simulink model "V2X_Core_SRI_coding_rate_symbol"  (R2023b)
settings: Solver=ode23tb  StartTime=0.0  StopTime=50  MaxStep=1e-2  RelTol=1e-3  AbsTol=1e-3
StopFcn:
  | run('saving.m')
values from neighbouring files (symbols this model uses):
  b = 1.6    [a2024_v2x_matlab_6veh.m]
  m = 2000    [a2024_v2x_matlab_6veh.m]
  mEgo = 1500    [a2024_v2x_matlab_6veh.m]
  Mode = 1    [a2024_v2x_matlab_6veh.m]    (also in v2x_matlab.m; v2x_matlabV2.m; v2x_matlab_6veh.m; v2x_matlab_R.m)
  RefSpeed = 90/3.6    (= 25)    [v2x_matlabV2.m]    (also in v2x_matlab_R.m)
  RelDistThreshold = 300    [v2x_matlabV2.m]    (also in v2x_matlab_R.m)
  s = RandStream("dsfmt19937","Seed",15)    [v2x_matlab.m]
  sampleTime = 0.1    [a2024_v2x_matlab_6veh.m]    (also in v2x_matlab.m; v2x_matlabV2.m; v2x_matlab_6veh.m; v2x_matlab_R.m)
  waypoints = [egoWP(:,2) egoWP(:,1), zeroforwp]    [a2024_v2x_matlab_6veh.m]    (also in misc.m = data.data.ActorSpecifications(1,1).Waypoints(:,[1,2]); v2x_matlab.m = data.data.ActorSpecifications(1,1).Waypoints(:,[1,2]); v2x_matlabV2.m = [5 -1.6 0; v2x_matlab_R.m = [5 -1.6 0)
  ZeroActors = struct(     'ActorID',0,     'Position', [1000 1000 1000],      'Velocity', [0 0 0],      'Roll', 0,      'Pitch', 0,      'Yaw', 0,      'AngularVelocity', [0 0 0])    [v2x_matlabV2.m]    (also in v2x_matlab_R.m)
undefined symbols (not defined in the file or in its folder): Battery, Brakes, Control, DiscIntNeverNeededParam, doppler, Drivetrain, ElectricMotor, Env, FB_flag, Init, SNR_value_list, Vehicle, Wheels
libraries: simulink x45, commofdm x29, commdigbbndam3 x15, commchan3 x14, simulink_extras x13, commcnvcod2 x12, commdigbbndpm3 x11, commblkintrlv2 x10, dspmathops x6, sharedtransform x6, autolibutils x6, autolibsharedcoupling x4
(part 2 of 8)

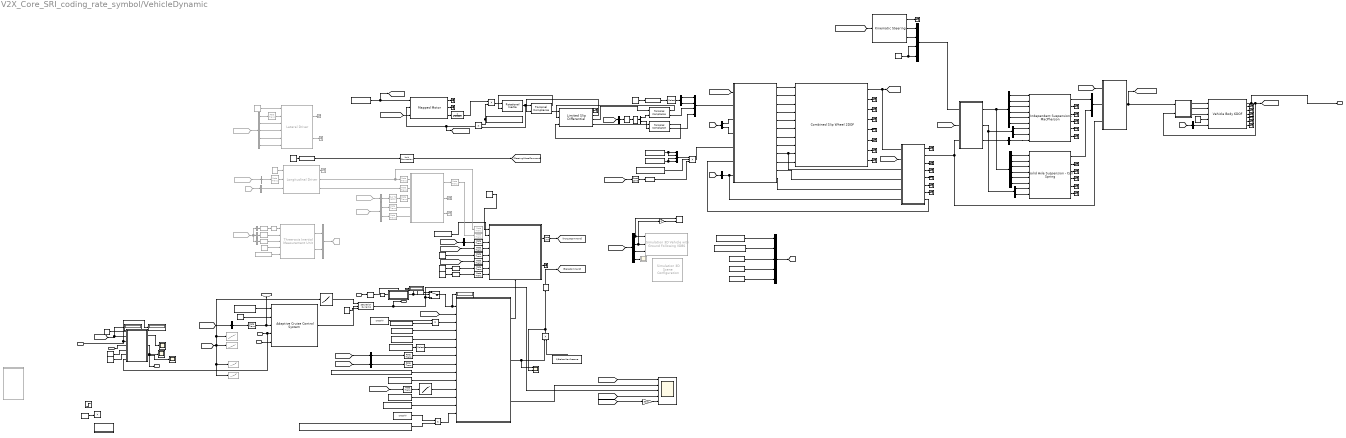
== system V2X_Core_SRI_coding_rate_symbol/VehicleDynamic ==
  note: ACC
  note: ENVIRONMENT
  note: CHASSIS
  note: VISAULS
  note: DRIVER INPUT
  note: WHEELS
  note: SUSPENSION
  note: STEERING
  note: ELECTRIC
  note: SENSOR
  note: BRAKE HYDRAULICS
  note: CONTROL
  note: DRIVETRAIN
  note: SRI
  u : Inport
  PDR : Inport  Port=2
  RelDist : Inport  Port=3
  RelativeVelocity : Inport  Port=4
  TTC : Inport  Port=5
  1-D Lookup Table : Lookup_n-D  NumberOfTableDimensions=1  BreakpointsForDimension1=ElectricMotor.SpeedVector  Table=ElectricMotor.TorqueVector  InternalRulePriority=Speed  RndMeth=Simplest
  1-D Lookup Table1 : Lookup_n-D  NumberOfTableDimensions=1  BreakpointsForDimension1=[0;5;15]  Table=[1;1.2;4]  InternalRulePriority=Speed  RndMeth=Simplest
  AccelerationToTrq : Subsystem
  Adaptive Cruise Control System1 : mpcadaslib/Adaptive Cruise Control System  EgoModel=tf([0.335,0.5],[0.3,0.7,0])  InitialEgoVelocity=Init.VelocityVector(1)  DefaultSpacing=10  MaxVelocity=60  MinAcceleration=-2  amin_ext=off  MaxAcceleration=4  amax_ext=off  Ts=0.1  PredictionHorizon=50  ControllerBehavior=0.950  suboptimal=off  maxiter=10  datatypeopt=double  optmode=off  trackmode=off
      settings: LibrarySourceBlock=mpclib/Automated Driving/Adaptive Cruise Control System
  Bus Creator : BusCreator  Inputs=2
  Bus Creator1 : BusCreator  Commented=on  Inputs=2
  Bus Creator2 : BusCreator  Inputs=5
  Bus Selector : BusSelector  OutputSignals=Front.zFront,Front.ReFront,Front.zdotFront,Front.FxFront,Front.FyFront,Front.MFront
  Bus Selector1 : BusSelector  Commented=on  OutputSignals=Omega,BrkPrs
  Bus Selector10 : BusSelector  OutputSignals=Omega
  Bus Selector11 : BusSelector  OutputSignals=BdyFrm.Cg.Vel.xdot
  Bus Selector12 : BusSelector  OutputSignals=Ground,Friction
  Bus Selector13 : BusSelector  OutputSignals=DCM
  Bus Selector14 : BusSelector  OutputSignals=WindXYZ
  Bus Selector15 : BusSelector  OutputSignals=InertFrm.Cg.Disp.X,InertFrm.Cg.Disp.Y,InertFrm.Cg.Ang.psi,BdyFrm.Cg.Vel.xdot
  Bus Selector16 : BusSelector  Commented=on  OutputSignals=Grade
  Bus Selector17 : BusSelector  Commented=on  OutputSignals=BdyFrm.Cg.Vel.xdot
  Bus Selector18 : BusSelector  Commented=on  OutputSignals=BdyFrm.Cg.Vel.xdot,InertFrm.Cg.Disp.Y,BdyFrm.Cg.Vel.ydot,InertFrm.Cg.Ang.psi,BdyFrm.Cg.AngVel.r
  Bus Selector19 : BusSelector  OutputSignals=BdyFrm.Cg.Vel.xdot
  Bus Selector2 : BusSelector  Commented=on  OutputSignals=BdyFrm.Cg.Acc.ax,BdyFrm.Cg.Acc.ay,BdyFrm.Cg.Acc.az  OutputAsBus=on
  Bus Selector20 : BusSelector  OutputSignals=Mx  OutputAsBus=on
  Bus Selector21 : BusSelector  OutputSignals=BdyFrm.Forces.Drag.Fx
  Bus Selector3 : BusSelector  OutputSignals=Front.VehPFront,Front.VehVFront
  Bus Selector4 : BusSelector  OutputSignals=Rear.VehPRear,Rear.VehVRear
  Bus Selector5 : BusSelector  Commented=on  OutputSignals=BdyFrm.Cg.AngVel.p,BdyFrm.Cg.AngVel.q,BdyFrm.Cg.AngVel.r  OutputAsBus=on
  Bus Selector6 : BusSelector  Commented=on  OutputSignals=BdyFrm.Cg.AngAcc.pdot,BdyFrm.Cg.AngAcc.qdot,BdyFrm.Cg.AngAcc.rdot  OutputAsBus=on
  Bus Selector7 : BusSelector  OutputSignals=Rear.zRear,Rear.ReRear,Rear.zdotRear,Rear.FxRear,Rear.FyRear,Rear.MRear
  Bus Selector8 : BusSelector  Commented=on  OutputSignals=BdyFrm.Cg.Acc.xddot,BdyFrm.Cg.Acc.yddot,BdyFrm.Cg.Acc.zddot  OutputAsBus=on
  Bus Selector9 : BusSelector  OutputSignals=StrgAngFront
  Bus to Vector{,1..3} (4 alike) : BusToVector  Commented=on
  Clock : simulink_extras/Flip Flops/Clock  period=sampleTime
  Combined Slip Wheel 2DOF : vehdynlibtire/Combined Slip Wheel 2DOF  tireType=Light passenger car 205/60R15  BrakeType=Disc  vertType=Magic Formula  plySteer=off  turnslip=off  mu_static=ones(1,4) .* Brakes.StaticFrictionCoeff  mu_kinetic=ones(1,4) .* Brakes.KineticFrictionCoeff  disk_abore=ones(1,4) .* Brakes.DiskBore  Rm=ones(1,4) .* Brakes.BrakePadMeanRadius  num_pads=ones(1,4) .* Brakes.NumPads  drum_abore=0.0508  drum_a=0.123  drum_c=0.212  drum_r=0.15  drum_theta1=0  drum_theta2=126  brake_p_bpt=[1 11.4736842105263 21.9473684210526 32.4210526315789 42.8947368421053 53.3684210526316 63.8421052631579 74.3157894736842 84.7894736842105 95.2631578947368 105.736842105263 116.210526315789 126.684210526316 137.157894736842 147.631578947368 158.105263157895 168.578947368421 179.052631578947 189.526315789474 200]  brake_n_bpt=[0 52.6315789473684 105.263157894737 157.894736842105 210.526315789474 263.157894736842 315.789473684211 368.421052631579 421.052631578947 473.684210526316 526.315789473684 578.947368421053 631.578947368421 684.210526315789 736.842105263158 789.473684210526 842.105263157895 894.736842105263 947.368421052632 1000]  f_brake_t=[43.4900602404453 42.5056030554862 41.5350898940194 40.5780454442085 39.6340111501808 38.7025443887544 37.7832176914519 36.8756180088306 35.9793460143796 35.0940154454303 34.2192524787115 33.3546951383474 32.4999927342521 31.6548053290159 30.8188032315107 29.991666515561 29.1730845621415 28.362755623661 27.5603864089927 26.765691687993;498.991217495636 487.695866636631 476.560505099801 465.579679307235 454.748127933653 444.060772460445 433.51270824929 423.099196101319 412.81565427025 402.657650900201 392.620896861006 382.701238955775 372.894653477208 363.197240090814 353.605216024701 344.114910546964 334.722759712992 325.425301366216 316.219170376863 307.10109410434;954.492374750826 932.886130217776 911.585920305583 890.581313170261 869.862244717126 849.419000532136 829.242198807128 809.322774193808 789.651962526121 770.221286354971 751.0225412433 732.047782773203 713.289314220164 694.739674852612 676.391628817892 658.238154578366 640.272434863842 622.48784710877 604.877954344734 587.436496520688;1409.99353200602 1378.07639379892 1346.61133551136 1315.58294703329 1284.9763615006 1254.77722860383 1224.97168936497 1195.5463522863 1166.48827078199 1137.78492180974 1109.42418562559 1081.39432659063 1053.68397496312 1026.28210961441 999.178041611083 972.361398609768 945.822110014692 919.550392851325 893.536738312604 867.771898937035;1865.49468926121 1823.26665738007 1781.63675071715 1740.58458089631 1700.09047828407 1660.13545667552 1620.7011799228 1581.76993037878 1543.32457903786 1505.34855726451 1467.82583000789 1430.74087040806 1394.07863570608 1357.82454437621 1321.96445440427 1286.48464264117 1251.37178516554 1216.61293859388 1182.19552228048 1148.10730135338;2320.9958465164 2268.45692096121 2216.66216592293 2165.58621475934 2115.20459506754 2065.49368474721 2016.43067048064 1967.99350847127 1920.16088729373 1872.91219271928 1826.22747439018 1780.08741422549 1734.47329644903 1689.36697913801 1644.75086719747 1600.60788667257 1556.92146031639 1513.67548433643 1470.85430624835 1428.44270376973;2776.49700377159 2713.64718454235 2651.68758112871 2590.58784862237 2530.31871185102 2470.8519128189 2412.16016103848 2354.21708656376 2296.9971955496 2240.47582817405 2184.62911877248 2129.43395804292 2074.86795719199 2020.9094138998 1967.53727999066 1914.73113070398 1862.47113546724 1810.73803007899 1759.51309021622 1708.77810618608;3231.99816102678 3158.8374481235 3086.71299633449 3015.58948248539 2945.43282863449 2876.21014089059 2807.88965159632 2740.44066465625 2673.83350380547 2608.03946362882 2543.03076315477 2478.78050186034 2415.26261793494 2352.4518486616 2290.32369278385 2228.85437473538 2168.02081061809 2107.80057582154 2048.17187418409 1989.11350860242;3687.49931828197 3604.02771170464 3521.73841154027 3440.59111634842 3360.54694541796 3281.56836896228 3203.61914215416 3126.66424274874 3050.66981206134 2975.60309908359 2901.43240753707 2828.12704567777 2755.6572786779 2683.9942834234 2613.11010557704 2542.97761876678 2473.57048576894 2404.8631215641 2336.83065815196 2269.44891101877;4143.00047553716 4049.21797528579 3956.76382674606 3865.59275021144 3775.66106220143 3686.92659703397 3599.34863271199 3512.88782084123 3427.50612031721 3343.16673453836 3259.83405191936 3177.4735894952 3096.05193942085 3015.5367181852 2935.89651837023 2857.10086279818 2779.12016091979 2701.92566730665 2625.48944211983 2549.78431343512;4598.50163279235 4494.40823886693 4391.78924195184 4290.59438407447 4190.77517898491 4092.28482510566 3995.07812326983 3899.11139893372 3804.34242857308 3710.73036999313 3618.23569630166 3526.82013331263 3436.44660016381 3347.079152947 3258.68293116342 3171.22410682959 3084.66983607064 2998.98821304921 2914.1482260877 2830.11971585147;5054.00279004754 4939.59850244808 4826.81465715762 4715.59601793749 4605.88929576838 4497.64305317735 4390.80761382767 4285.3349770262 4181.17873682896 4078.2940054479 3976.63734068395 3876.16667713006 3776.84126090677 3678.62158770879 3581.46934395661 3485.34735086099 ...(+2764 chars)]  tireParamSet=vdynPassCar.mat  PRESMAX=Wheels.MaxPressure  PRESMIN=Wheels.MinPressure  FZMAX=Wheels.MaxForceZ  FZMIN=Wheels.MinForceZ  VXLOW=Wheels.VelocityTolelranceLow  KPUMAX=Wheels.MaxSlipRatio  KPUMIN=Wheels.MinSlipRatio  ALPMAX=Wheels.MaxSlipAngle  ALPMIN=Wheels.MinSlipAngle  CAMMAX=Wheels.MaxCamber  CAMMIN=Wheels.MinCamber  LONGVL=Wheels.NomLongSpd  FxRelFreqLwrLim=200*pi  FyRelFreqLwrLim=50*pi  MyRelFreqLwrLim=50*pi  omegao=(Init.VelocityVector(1) / Wheels.EffectiveRadius) * ones(1,4)  br=Wheels.RotationalDamping  UNLOADED_RADIUS=Wheels.UnloadedRadius  NOMPRES=Wheels.NominalPressure  FNOMIN=Wheels.NominalForceZ  WIDTH=Wheels.WheelWidth  RIM_RADIUS=Wheels.RimRadius  MASS=Wheels.Mass  IYY=Wheels.RotationalInertia  GRAVITY=Env.Gravity  zo=-Init.PositionVector(3).*ones(1,4)  zdoto=zeros(1,4)  BREFF=8.25094594147963  DREFF=0.260468730454265  FREFF=0.0735298544471851  Q_RE0=1.00866439868088  Q_V1=0.000760413786224011  Q_V2=0.0463384792019201  Q_FZ1=0  Q_FZ2=15.6870832810226  Q_FZ3=0  Q_FCX=0.138643970247602  Q_FCY=0.10843499565426  Q_FCY2=-0.465763352339538  PFZ1=0.69958166705601  VERTICAL_STIFFNESS=207885.061134007  VERTICAL_DAMPING=ones(1,4).*500  BOTTOM_OFFST=0.00990653336182505  BOTTOM_STIFF=1999075.87051971  LONGITUDINAL_STIFFNESS=388714.175879854  LATERAL_STIFFNESS=157087.404633332  PCFX1=0.18539229191199  PCFX2=0  PCFX3=0  PCFY1=0.163183345037677  PCFY2=0  PCFY3=0.249094918231954  Q_RA1=0.675942571700787  Q_RA2=0.73800463546164  Q_RB1=1.04487486456705  Q_RB2=-1.191763806629  PCX1=1.58523057950359  PDX1=1.0239116238178  PDX2=-0.0842405110022724  PDX3=0  PEX1=0.110312777158455  PEX2=0.313468516038146  PEX3=0  PEX4=0.0016060905760045  PKX1=21.3872544684023  PKX2=14.0006541873175  PKX3=-0.405326109653452  PHX1=0.000212599305364818  PHX2=0.00115950515263055  PVX1=1.59236164471432e-05  PVX2=0.000104321112127671  PPX1=-0.349461321276586  PPX2=0.387840040616429  PPX3=-0.0969947336569324  PPX4=0.0632271859795801  RBX1=12.7633329850276  RBX2=9.5787123658471  RBX3=0  RCX1=1.02796280922059  REX1=-0.45202516851367  REX2=-0.47304886171176  RHX1=0.000233272373115809  QSX1=-0.00788307788961443  QSX2=0.954629515459396  QSX3=0.0155855777667025  QSX4=0.125904607142414  QSX5=1.01110069703963  QSX6=20.1938577118433  QSX7=0.310818120717083  QSX8=-0.0430823751139655  QSX9=0.636494404888216  QSX10=0.142438060591663  QSX11=0.346766530036373  QSX12=0  QSX13=0  QSX14=0  PPMX1=0  PCY1=1.34299950037631  PDY1=0.878267729082195  PDY2=-0.0644597923147385  PDY3=0  PEY1=-0.809776534470972  PEY2=-0.600180598867198  PEY3=0.0991732552633487  PEY4=-6.5577974035573  PEY5=0  PKY1=-15.5714726518315  PKY2=1.73126522291751  PKY3=0.365349873517229  PKY4=1.98176755955416  PKY5=0  PKY6=-0.884005199550313  PKY7=-0.237259727611847  PHY1=-0.00183370557235628  PHY2=0.00346401302716671  PVY1=-0.00675427560163264  PVY2=0.036379218103843  PVY3=-0.163543984089166  PVY4=-0.491003349625726  PPY1=-0.62059646553185  PPY2=-0.0647824842338686  PPY3=-0.164648843290686  PPY4=0.283193909060098  PPY5=0  RBY1=10.7588809173639  RBY2=7.70420065295029  RBY3=3.40283755070691e-06  RBY4=0  RCY1=1.06691874059059  REY1=0.308244924574305  REY2=7.48775032604508e-06  RHY1=0.0118479204960415  RHY2=7.63650177161071e-06  RVY1=0.0560024425050078  RVY2=7.48487127056197e-06  RVY3=0  RVY4=98.4047026517149  RVY5=2.02759273900054  RVY6=15.7623064923347  QSY1=0.00699077564863536  QSY2=0  QSY3=0.00153535478298811  QSY4=8.55710322455322e-05  QSY5=0  QSY6=0  QSY7=0.89443879773793  QSY8=-0.403227641260894  QBZ1=11.666656027484  QBZ2=-1.30355438574485  QBZ3=0  QBZ4=0.177918305399071  QBZ5=-0.162481135068033  QBZ6=0  QBZ9=30.1445534682089  QBZ10=0  QCZ1=1.29026978207574  QDZ1=0.0886972644991399  QDZ2=-0.0058634820161856  QDZ3=0.3805597481383  QDZ4=0  QDZ6=0.00160914918118959  QDZ7=-0.00211036330862154  QDZ8=-0.13921904912557  QDZ9=0.00816585550028243  QDZ10=0  QDZ11=0  QEZ1=-2.19802254534746  QEZ2=1.01850535789165  QEZ3=0  QEZ4=0.278379679112054  QEZ5=-0.548414722765386  QHZ1=0.00148361198869669  QHZ2=0.00202017567585904  QHZ3=0.240316641332066  QHZ4=-0.210114035738085  PPZ1=-0.443927982388615  PPZ2=0  SSZ1=0.00914999585397887  SSZ2=0.0389830656052735  SSZ3=0  SSZ4=0  PDXP1=0.396718274678791  PDXP2=0  PDXP3=0  PKYP1=1.00587060633573  PDYP1=0.40483048923438  PDYP2=0  PDYP3=0  PDYP4=0  PHYP1=0.992731942067188  PHYP2=0.150352945499914  PHYP3=0  PHYP4=-3.98988682633674  PECP1=0.502379254513503  PECP2=0  QDTP1=10.0178654287947  QCRP1=0.200627747200702  QCRP2=0.0995735881599772  QBRP1=0.0997107127960717  QDRP1=1.01432910167423  QDRP2=0  aMode=2
  Compare To Constant1 : simulink/Logic and Bit Operations/Compare To Constant  relop=<=  const=FB_flag  OutDataTypeStr=boolean
  Constant{,13,18,29,35,38} (6 alike) : Constant  Value=0
  Constant1 : Constant  Value=[0;0;0]
  Constant10 : Constant  Commented=on  Value=[0,0,Env.Gravity]
  Constant11 : Constant  Commented=on  Value=10
  Constant12 : Constant  Commented=on  Value=Init.PositionVector(2)
  Constant14 : Constant  Value=repmat(eye(3), 1, 1,4)
  Constant15 : Constant  Value=ones(1,4).*0.8
  Constant16 : Constant  Value=zeros(1,4)
  Constant17 : Constant  Value=zeros(1,3)
  Constant19 : Constant  Value=RefSpeed
  Constant2 : Constant  Value=Brakes.BiasFront
  Constant20 : Constant  Value=1.4
  Constant21 : Constant  Value=1/Brakes.MaxPressure
  Constant22 : Constant  Value=-2
  Constant23 : Constant  Value=Wheels.RotationalInertia
  Constant24 : Constant  Value=Wheels.UnloadedRadius
  Constant25 : Constant  Value=Vehicle.Mass
  Constant26 : Constant  Value=ElectricMotor.Inertia
  Constant27 : Constant  Value=Drivetrain.EngineToRearDriveshaftRatio*Drivetrain.RearDifferential.CarrierToDriveshaftRatio
  Constant28 : Constant
  Constant3 : Constant  Value=Brakes.BiasRear
  Constant30 : Constant  Value=ones(4)
  Constant31 : Constant  Value=zeros(4,1)
  Constant32 : Constant  Value=Brakes.KineticFrictionCoeff*pi*Brakes.DiskBore^2*Brakes.BrakePadMeanRadius*Brakes.NumPads/4
  Constant33 : Constant  Value=Brakes.MaxPressure
  Constant34 : Constant  Value=-9.81
  Constant36 : Constant  Value=ones(4)
  Constant37 : Constant  Value=Drivetrain.EngineToRearDriveshaftRatio
  Constant39 : Constant  Value=0.1
  Constant4 : Constant  Value=ones(1,4).*Brakes.MaxPressure
  Constant40 : Constant  Value=90/3.6
  Constant41 : Constant
  Constant5 : Constant  Value=Battery.IdealVoltage  SampleTime=-1
  Constant6 : Constant  Value=0.8  SampleTime=-1
  Constant7 : Constant  Value=-525  SampleTime=-1
  Constant8 : Constant  Value=525  SampleTime=-1
  Constant9 : Constant  Commented=on  Value=[0,0,0]
  Dead Zone : DeadZone  LowerValue=-inf  UpperValue=1e-3  ZeroCross=off
  Demux1 : Demux  Outputs=2
  Demux2 : Demux  Outputs=2
  Display{,1..3} (4 alike) : Display
  Driveshaft Compliance : autolibsharedcoupling/Torsional Compliance  port_config=Simulink  extInfo=off  k=Drivetrain.RearDriveshaft.TorsionalStiffness  b=Drivetrain.RearDriveshaft.TorsionalDamping  theta_o=Init.RearDriveshaftDeflection  domega_o=Init.RearDriveshaftVelocityDifference  omega_c=Drivetrain.RearDriveshaft.DampingCuroffFreq  blkID=0  aMode=1
  DrivetrainControlUnit : Subsystem
      settings: PortSchema="{\"entries\":[{\"content\":{\"sides\":[{\"content\":{\"connectorIds\":[\"In1\",\"In2\",\"In3\",\"In4\",\"In5\",\"In6\",\"In7\",\"In8\"]},\"type\":\"ConnectorPlacement.EquallySpacedRectSide\",\"uuid\":\"dbe5afd4-97c8-4fc8-af85-c2807fe6ed52\"},{\"content\":{\"connectorIds\":[\"Out1\",\"Out2\"],\"side\":\"RIGHT\"},\"type\":\"ConnectorPlacement.EquallySpacedRectSide\",\"uuid\":\"42ecce8e-1af3-4fa4-ab97-a4ae9e0c6691\"},{\"content\":{\"side\":\"TOP\"},\"type\":\"ConnectorPlacement.EquallySpacedRectSide\",\"uuid\":\"ed6d3e7b-a7c7-4819-a691-619a2b8297d4\"},{\"content\":{\"connectorIds\":[\"In9\"],\"side\":\"BOTTOM\"},\"type\":\"ConnectorPlacement.EquallySpacedRectSide\",\"uuid\":\"6ce4a012-6abe-4502-ba9b-cc2ba462b8c5\"}]},\"type\":\"ConnectorPlacement.EquallySpacedConnector\",\"uuid\":\"8ef0b83d-6ce0-4cb9-a7c1-79ef86bbfb87\"}],\"packageUris\":[\"http://schema.mathworks.com/mf0/Connector/R2020b\"],\"version\":\"1.0\"}"
  Enabled Subsystem : Subsystem  TreatAsAtomicUnit=on
  First Order Hold : FirstOrderHold  ErrorTolerance=1e-3  AllowContinuousInput=on
  FiveSteteABS-TCS : Subsystem  Commented=on
  From{11,18..20} (4 alike) : From  Commented=on  GotoTag=VehicleFbdk
  From17 : From  Commented=on  GotoTag=ENV
  From5 : From  Commented=on  GotoTag=WheelFbdk
  Gain : Gain  Gain=-1
  Gain1 : Gain  Gain=30/pi
  Goto6 : Goto  Commented=on  GotoTag=IMU
  Kinematic Steering : vehdynlibsteering/Kinematic Steering  StrgType=Ackerman  StrgRatioType=Constant  Loc=Front  NrmlFctr=0.01  TrckWdth=Vehicle.TrackWidthFront  WhlBase=Vehicle.CG.LongDistFrontAxle + Vehicle.CG.LongDistRearAxle  Db=0  StrgRng=Steering.SteerRange  StrgAngBpts="[-6.2832   -5.0265   -3.7699   -2.5133   -1.2566         0    1.2566    2.5133    3.7699    5.0265    6.2832]"  StrgRatioTbl=|  StrgRatio=Steering.SteeringRatio  PctAckIn=off  PctAck=100  PctAckTbl=ones(1,11)*100  StrgArmLngth=0.1  RckCsLngth=0.5  TieRodLngth=0.248  D=0.2  PnnRadius=0.00085818  PnnRadiusTbl="[0.0055    0.0055    0.0056    0.0057    0.0058    0.0057    0.0057    0.0057    0.0056    0.0055    0.0055]"  RodLngth=0.1  ParaArmLngth=0.9  aMode=2
      | [13.5000   13.3750   13.2500   13.1250   13.0000   13.0000   13.0000   13.1250   13.2500   13.3750   13.5000
      | ]
  Lateral Driver : vehdynlibdriver/Lateral Driver  Commented=on  extSteerOvr=off  extSteerHld=off  extSteerZero=off  steerOut=on  cntrlTypeLat=Predictive  coordMode=SAE J670 (Z-down)  angUnits=rad  tau=0.1  L=3  vecPose=off  dynamMode=off  PositionGainF=2.5  PositionGainR=2.5  YawRateGain=.2  DelayGain=.2  a=Vehicle.CG.LongDistFrontAxle  b=Vehicle.CG.LongDistRearAxle  m=Vehicle.Mass  Cy_f=25266  Cy_r=70933  I=Vehicle.InertiaYaw  Ksteer=18  theta=45*pi/180  aMode=2
  Limited Slip Differential : autolibshareddiff/Limited Slip Differential  DiffEffModelPopup=Constant  InterpMethod=Linear point-slope  extTamb=off  shaftSwitchMask=To the left of center-line  Ndiff=Drivetrain.RearDifferential.CarrierToDriveshaftRatio  Jd=Drivetrain.RearDifferential.CarrierInertia  bd=Drivetrain.RearDifferential.CarrierDamping  Jw1=Drivetrain.RearDifferential.AxleLeftInertia  bw1=Drivetrain.RearDifferential.AxleLeftDamping  Jw2=Drivetrain.RearDifferential.AxleRightInertia  bw2=Drivetrain.RearDifferential.AxleRightDamping  omegaw1o=Init.VelocityVector(1) / Wheels.EffectiveRadius  omegaw2o=Init.VelocityVector(1) / Wheels.EffectiveRadius  eta=Drivetrain.RearDifferential.EfficiencyFactor  eta_tbl=reshape([0.64 0.76 0.8 0.81 0.83 0.84 0.84 0.56 0.73 0.78 0.8 0.83 0.84 0.84 0.54 0.71 0.77 0.8 0.82 0.84 0.84 0.53 0.71 0.77 0.8 0.83 0.84 0.84 0.51 0.71 0.77 0.8 0.83 0.84 0.85 0.52 0.7 0.77 0.8 0.83 0.84 0.85 0.51 0.71 0.76 0.79 0.83 0.84 0.85 0.5 0.69 0.76 0.79 0.82 0.84 0.85 0.45 0.68 0.75 0.78 0.82 0.84 0.85 0.43 0.67 0.74 0.78 0.81 0.83 0.84 0.38 0.63 0.71 0.75 0.8 0.82 0.83 0.81 0.86 0.88 0.89 0.89 0.89 0.9 0.77 0.85 0.87 0.88 0.89 0.9 0.9 0.72 0.82 0.86 0.87 0.88 0.89 0.9 0.68 0.8 0.84 0.86 0.88 0.89 0.89 0.67 0.8 0.84 0.86 0.88 0.89 0.9 0.67 0.8 0.84 0.86 0.88 0.89 0.9 0.65 0.8 0.84 0.86 0.88 0.89 0.9 0.64 0.79 0.83 0.86 0.88 0.89 0.9 0.63 0.78 0.83 0.86 0.88 0.89 0.9 0.59 0.76 0.82 0.85 0.87 0.89 0.9 0.53 0.73 0.8 0.83 0.86 0.88 0.89], 7, 11, 2)  Trq_bpts=[25, 50, 75, 100, 150, 200, 250]  omega_bpts=[52.4 78.5 105 131 157 183 209 262 314 419 524]  Temp_bpts=[290 358]  Tamb=297.15  couplingType=Pre-loaded ideal clutch  Ndisks=Drivetrain.RearDifferential.ClutchNumDisk  Reff=Drivetrain.RearDifferential.ClutchEffRadius  Fc=Drivetrain.RearDifferential.ClutchPreloadForce  muc=Drivetrain.RearDifferential.ClutchFrictionCoeffVector  dw=Drivetrain.RearDifferential.ClutchSlipSpeedVector  Tdw=[-100, -90, -50, -5, 0, 5, 50, 90, 100]  dwT=[-200, -175, -100, - 50, 0, 50, 100, 175, 200]  TTin=[-200 -175 -100 - 50 0 50 100 175 200]  Tin=[-200 -175 -100 - 50 0 50 100 175 200]  tauC=Drivetrain.RearDifferential.ClutchCouplingTimeConstant  IdealInterpMethod=Linear point-slope  IdealExtrapMethod=Clip  TdwInterpMethod=Linear point-slope  TdwExtrapMethod=Clip  TTinInterpMethod=Linear point-slope  TTinExtrapMethod=Clip  maxAbsSpd=5e3  aMode=1
      settings: LibrarySourceBlock=autolibdiff/Limited Slip Differential
  Longitudinal Driver : autolibshared/Longitudinal Driver  Commented=on  extAccelOvr=off  extDecelOvr=off  extAccelHld=off  extDecelHld=off  extAccelZero=off  extDecelZero=off  cntrlType=PI  shftType=None  velUnits=m/s  gearOut=off  Kp=15  Ki=1  Kff=.05  Kg=.01  VehVelVec=[0 100]  KffVec=[.1 .1]  KpVec=[10 10]  KiVec=[5 5]  KgVec=[0 0]  m=1500  Kpt=3000  tau=.1  L=2  aR=200  bR=2.5  cR=.5  g=9.81  vnom=100  Kaw=.1  tauerr=.03  tauPt=2  GearInit=0  tShift=.1  pdlVec=[0.1 0.4 0.5 0.9]  upShftTbl=[-1 12.9375 26.4375 39.9375 51.18749999999999 62.4375 72.84375 83.25;-1 16.3125 29.8125 43.3125 54.5624 65.8125 76.78125 87.75;-1 19.6875 33.1875 46.68749999999999 57.9375 69.1875 80.71875 92.25;-1 33 52.5 77.25 100.5 138.75 161.875 185]  dwnShftTbl=[1 9.5625 23.0625 36.5625 47.8125 59.0625 68.90625 78.75;1 12.9375 26.4375 39.9375 51.18749999999999 62.4375 72.84375 83.25;1 16.3125 29.8125 43.3125 54.562499 65.8125 76.78125 87.75;1 19.6875 33.1875 46.68749999999999 57.9375 69.1875 80.71875 92.25]  tClutch=.5  tRev=.5  tPark=120  aMode=1  UpGearVec="[0  1  2  3  4  5  6  7]"  DownGearVec="[1  2  3  4  5  6  7  8]"
  MATLAB Function1 : MATLAB Function  TreatAsAtomicUnit=on
  MATLAB Function2 : MATLAB Function  Commented=on  TreatAsAtomicUnit=on
  Mapped Motor : autolibmappedmotor/Mapped Motor  port_config=Speed  param_by=Tabulated torque-speed envelope  w_t=ElectricMotor.SpeedVector  T_t=ElectricMotor.TorqueVector  torque_max=0.1  power_max=30  Tc=ElectricMotor.TorqueTimeConst  param_loss=Tabulated efficiency data  eff=100  w_eff=375  T_eff=0.08  Piron=0  Pbase=0  w_eff_bp=ElectricMotor.SpeedVector  T_eff_bp=ElectricMotor.TorqueEfficiencyVector  Temp_eff_bp=Temp_eff_bp  losses_table=PlntEM1TrqLossTbl  losses_table_3d=losses_table_3d  efficiency_table=ElectricMotor.EfficiencyTable  efficiency_table_3d=efficiency_table_3d  J=5e-6  b=1e-5  omega_o=0  T_t_extended=[125.931348721462 137.379653150686 151.117618465755 167.90846496195 188.897023082193 215.882312093935 251.862697442924 302.235236931509 377.794046164387 450 450 450 450 450 450 450 450 450 377.794046164387 302.235236931509 251.862697442924 215.882312093935 188.897023082193 167.90846496195 151.117618465755 137.379653150686 125.931348721462]  w_t_extended=[-1675.51608191456 -1535.88974175501 -1396.26340159546 -1256.63706143592 -1117.01072127637 -977.384381116825 -837.758040957278 -698.131700797732 -558.505360638185 -468.888888888889 -418.879020478639 -279.252680319093 -139.626340159546 0 139.626340159546 279.252680319093 418.879020478639 468.888888888889 558.505360638185 698.131700797732 837.758040957278 977.384381116825 1117.01072127637 1256.63706143592 1396.26340159546 1535.88974175501 1675.51608191456]  KLossIron=0  KLossCopper=0  x_w_eff_vec=[-1675.51608191456 -1535.88974175501 -1396.26340159546 -1256.63706143592 -1117.01072127637 -977.384381116825 -837.758040957278 -698.131700797732 -558.505360638185 -468.888888888889 -418.879020478639 -279.252680319093 -139.626340159546 0 139.626340159546 279.252680319093 418.879020478639 468.888888888889 558.505360638185 698.131700797732 837.758040957278 977.384381116825 1117.01072127637 1256.63706143592 1396.26340159546 1535.88974175501 1675.51608191456]  x_T_eff_vec=[-450 -405 -360 -315 -270 -225 -180 -135 -90 -45 0 45 90 135 180 225 270 315 360 405 450]  x_tmp_eff_vec=[233.15 293.15 373.15]  x_losses_mat=[56751.351161622 51076.2160454598 45401.0809292976 39725.9458131354 34050.8106969732 28375.675580811 22700.5404646488 17025.4053484866 14913.9343555032 12274.1294372811 0 10555.7513160617 13571.6802635079 15833.6269740925 21111.5026321234 26389.3782901542 31667.2539481851 36945.1296062159 42223.0052642468 47500.8809222776 52778.7565803085;52022.0718981535 46819.8647083382 41617.6575185228 36415.4503287075 31213.2431388921 26011.0359490768 20808.8287592614 15606.6215694461 12020.0066746044 11251.2853175076 0 9676.10537305656 11058.4061406361 14514.1580595848 19352.2107461131 24190.2634326414 29028.3161191697 33866.3688056979 38704.4214922262 43542.4741787545 48380.5268652828;47292.792634685 42563.5133712165 37834.234107748 33104.9548442795 28375.675580811 23646.3963173425 18917.117053874 14187.8377904055 10927.2787950949 10228.4411977342 0 8796.45943005142 10053.0964914873 13194.6891450771 17592.9188601028 21991.1485751285 26389.3782901542 30787.60800518 35185.8377202057 39584.0674352314 43982.2971502571;42563.5133712165 38307.1620340949 34050.8106969732 29794.4593598516 25538.1080227299 21281.7566856083 17025.4053484866 12769.054011365 11185.4507666274 9205.59707796079 0 7916.81348704628 10178.7601976309 11875.2202305694 15833.6269740925 19792.0337176157 23750.4404611388 27708.847204662 31667.2539481851 35625.6606917082 39584.0674352314;37834.234107748 34050.8106969732 30267.3872861984 26483.9638754236 22700.5404646488 18917.117053874 15133.6936430992 11350.2702323244 9942.62290366878 8182.75295818737 0 7037.16754404114 9047.7868423386 10555.7513160617 14074.3350880823 17592.9188601028 21111.5026321234 24630.086404144 28148.6701761645 31667.2539481851 35185.8377202057;33104.9548442795 29794.4593598516 26483.9638754236 23173.4683909957 19862.9729065677 16552.4774221398 15298.1903131329 11473.6427348497 9773.84381116825 8377.58040957278 0 7037.16754404114 8796.45943005142 10555.7513160617 14074.3350880823 15393.80400259 18472.564803108 21551.325603626 24630.086404144 27708.847204662 30787.60800518;28375.675580811 25538.1080227299 22700.5404646488 19862.9729065677 17025.4053484866 16390.9181926424 14913.9343555032 11185.4507666274 10281.575957203 8275.41479482189 0 6785.84013175395 9047.7868423386 10178.7601976309 13571.6802635079 15079.644737231 15833.6269740925 18472.564803108 21111.5026321234 23750.4404611388 26389.3782901542;31070.6965739649 27963.6269165685 21854.5575901899 19122.7378914161 16390.9181926424 15535.3482869825 12428.278629586 10471.975511966 8567.97996433581 6896.17899568491 0 5654.86677646163 7539.8223686155 9424.77796076938 11309.7335529233 14137.1669411541 15079.644737231 17592.9188601028 20106.1929829747 25446.9004940773 28274.3338823081;34271.9198573432 30844.7278716089 27417.5358858746 19547.6876223365 16755.1608191456 13962.6340159546 11170.1072127637 10281.575957203 8182.75295818737 6283.18530717959 0 5026.54824574367 7037.16754404114 9047.78684233861 10053.0964914873 12566.3706143592 15079.644737231 17592.9188601028 24127.4315795696 27143.3605270158 30159.289474462;34348.8372093023 30913.9534883721 27479.0697674419 20140.9090909091 17263.6363636364 14386.3636363636 11509.0909090909 8631.81818181819 6869.76744186047 5275 0 4220 5908 7596 10128 12660 15192 17724 23632 26586 29540;35903.9160410262 32313.5244369236 24548.2588745621 21479.7265152418 15422.3639358044 12851.9699465037 10281.575957203 9205.59707796079 6137.06471864053 4712.38898038469 0 3769.91118430775 5277.87565803085 7916.81348704628 9047.7868423386 11309.7335529233 13571.6802635079 18472.564803108 21111.5026321234 27143.3605270158 30159.289474462;27584.7159827396 24826.2443844657 19148.7552218806 16755.1608191456 12274.1294372811 10228.4411977342 8182.75295818737 6137.06471864053 4787.18880547016 3544.36094251156 0 2764.60153515902 4021.23859659494 5277.87565803085 7037.16754404114 8796.45943005142 10555.7513160617 14074.3350880823 16084.9543863797 20357.5203952619 22619.4671058465;26927.9370307696 19868.4508362165 15873.3102497169 ...(+4614 chars)]  x_losses_mat_3d=cat(3,[2 2 2 2 2 2 2 2 2 2 2 2 2 2 2 2 2 2 2 2 2;2 2 2 2 2 2 2 2 2 2 2 2 2 2 2 2 2 2 2 2 2;2 2 2 2 2 2 2 2 2 2 2 2 2 2 2 2 2 2 2 2 2;2 2 2 2 2 2 2 2 2 2 2 2 2 2 2 2 2 2 2 2 2;2 2 2 2 2 2 2 2 2 2 2 2 2 2 2 2 2 2 2 2 2;2 2 2 2 2 2 2 2 2 2 2 2 2 2 2 2 2 2 2 2 2;2 2 2 2 2 2 2 2 2 2 2 2 2 2 2 2 2 2 2 2 2;2 2 2 2 2 2 2 2 2 2 2 2 2 2 2 2 2 2 2 2 2;2 2 2 2 2 2 2 2 2 2 2 2 2 2 2 2 2 2 2 2 2;2 2 2 2 2 2 2 2 2 2 2 2 2 2 2 2 2 2 2 2 2;2 2 2 2 2 2 2 2 2 2 2 2 2 2 2 2 2 2 2 2 2;2 2 2 2 2 2 2 2 2 2 2 2 2 2 2 2 2 2 2 2 2;2 2 2 2 2 2 2 2 2 2 2 2 2 2 2 2 2 2 2 2 2;2 2 2 2 2 2 2 2 2 2 2 2 2 2 2 2 2 2 2 2 2;2 2 2 2 2 2 2 2 2 2 2 2 2 2 2 2 2 2 2 2 2;2 2 2 2 2 2 2 2 2 2 2 2 2 2 2 2 2 2 2 2 2;2 2 2 2 2 2 2 2 2 2 2 2 2 2 2 2 2 2 2 2 2;2 2 2 2 2 2 2 2 2 2 2 2 2 2 2 2 2 2 2 2 2;2 2 2 2 2 2 2 2 2 2 2 2 2 2 2 2 2 2 2 2 2;2 2 2 2 2 2 2 2 2 2 2 2 2 2 2 2 2 2 2 2 2;2 2 2 2 2 2 2 2 2 2 2 2 2 2 2 2 2 2 2 2 2;2 2 2 2 2 2 2 2 2 2 2 2 2 2 2 2 2 2 2 2 2;2 2 2 2 2 2 2 2 2 2 2 2 2 2 2 2 2 2 2 2 2;2 2 2 2 2 2 2 2 2 2 2 2 2 2 2 2 2 2 2 2 2;2 2 2 2 2 2 2 2 2 2 2 2 2 2 2 2 2 2 2 2 2;2 2 2 2 2 2 2 2 2 2 2 2 2 2 2 2 2 2 2 2 2;2 2 2 2 2 2 2 2 2 2 2 2 2 2 2 2 2 2 2 2 2],[1.5 1.5 1.5 1.5 1.5 1.5 1.5 1.5 1.5 1.5 1.5 1.5 1.5 1.5 1.5 1.5 1.5 1.5 1.5 1.5 1.5;1.5 1.5 1.5 1.5 1.5 1.5 1.5 1.5 1.5 1.5 1.5 1.5 1.5 1.5 1.5 1.5 1.5 1.5 1.5 1.5 1.5;1.5 1.5 1.5 1.5 1.5 1.5 1.5 1.5 1.5 1.5 1.5 1.5 1.5 1.5 1.5 1.5 1.5 1.5 1.5 1.5 1.5;1.5 1.5 1.5 1.5 1.5 1.5 1.5 1.5 1.5 1.5 1.5 1.5 1.5 1.5 1.5 1.5 1.5 1.5 1.5 1.5 1.5;1.5 1.5 1.5 1.5 1.5 1.5 1.5 1.5 1.5 1.5 1.5 1.5 1.5 1.5 1.5 1.5 1.5 1.5 1.5 1.5 1.5;1.5 1.5 1.5 1.5 1.5 1.5 1.5 1.5 1.5 1.5 1.5 1.5 1.5 1.5 1.5 1.5 1.5 1.5 1.5 1.5 1.5;1.5 1.5 1.5 1.5 1.5 1.5 1.5 1.5 1.5 1.5 1.5 1.5 1.5 1.5 1.5 1.5 1.5 1.5 1.5 1.5 1.5;1.5 1.5 1.5 1.5 1.5 1.5 1.5 1.5 1.5 1.5 1.5 1.5 1.5 1.5 1.5 1.5 1.5 1.5 1.5 1.5 1.5;1.5 1.5 1.5 1.5 1.5 1.5 1.5 1.5 1.5 1.5 1.5 1.5 1.5 1.5 1.5 1.5 1.5 1.5 1.5 1.5 1.5;1.5 1.5 1.5 1.5 1.5 1.5 1.5 1.5 1.5 1.5 1.5 1.5 1.5 1.5 1.5 1.5 1.5 1.5 1.5 1.5 1.5;1.5 1.5 1.5 1.5 1.5 1.5 1.5 1.5 1.5 1.5 1.5 1.5 1.5 1.5 1.5 1.5 1.5 1.5 1.5 1.5 1.5;1.5 1.5 1.5 1.5 1.5 1.5 1.5 1.5 1.5 1.5 1.5 1.5 1.5 1.5 1.5 1.5 1.5 1.5 1.5 1.5 1.5;1.5 1.5 1.5 1.5 1.5 1.5 1.5 1.5 1.5 1.5 1.5 1.5 1.5 1.5 1.5 1.5 1.5 1.5 1.5 1.5 1.5;1.5 1.5 1.5 1.5 1.5 1.5 1.5 1.5 1.5 1.5 1.5 1.5 1.5 1.5 1.5 1.5 1.5 1.5 1.5 1.5 1.5;1.5 1.5 1.5 1.5 1.5 1.5 1.5 1.5 1.5 1.5 1.5 1.5 1.5 1.5 1.5 1.5 1.5 1.5 1.5 1.5 1.5;1.5 1.5 1.5 1.5 1.5 1.5 1.5 1.5 1.5 1.5 1.5 1.5 1.5 1.5 1.5 1.5 1.5 1.5 1.5 1.5 1.5;1.5 1.5 1.5 1.5 1.5 1.5 1.5 1.5 1.5 1.5 1.5 1.5 1.5 1.5 1.5 1.5 1.5 1.5 1.5 1.5 1.5;1.5 1.5 1.5 1.5 1.5 1.5 1.5 1.5 1.5 1.5 1.5 1.5 1.5 1.5 1.5 1.5 1.5 1.5 1.5 1.5 1.5;1.5 1.5 1.5 1.5 1.5 1.5 1.5 1.5 1.5 1.5 1.5 1.5 1.5 1.5 1.5 1.5 1.5 1.5 1.5 1.5 1.5;1.5 1.5 1.5 1.5 1.5 1.5 1.5 1.5 1.5 1.5 1.5 1.5 1.5 1.5 1.5 1.5 1.5 1.5 1.5 1.5 1.5;1.5 1.5 1.5 1.5 1.5 1.5 1.5 1.5 1.5 1.5 1.5 1.5 1.5 1.5 1.5 1.5 1.5 1.5 1.5 1.5 1.5;1.5 1.5 1.5 1.5 1.5 1.5 1.5 1.5 1.5 1.5 1.5 1.5 1.5 1.5 1.5 1.5 1.5 1.5 1.5 1.5 1.5;1.5 1.5 1.5 1.5 1.5 1.5 1.5 1.5 1.5 1.5 1.5 1.5 1.5 1.5 1.5 1.5 1.5 1.5 1.5 1.5 1.5;1.5 1.5 1.5 1.5 1.5 1.5 1.5 1.5 1.5 1.5 1.5 1.5 1.5 1.5 1.5 1.5 1.5 1.5 1.5 1.5 1.5;1.5 1.5 1.5 1.5 1.5 1.5 1.5 1.5 1.5 1.5 1.5 1.5 1.5 1.5 1.5 1.5 1.5 1.5 1.5 1.5 1.5;1.5 1.5 1.5 1.5 1.5 1.5 1.5 1.5 1.5 1.5 1.5 1.5 1.5 1.5 1.5 1.5 1.5 1.5 1.5 1.5 1.5;1.5 1.5 1.5 1.5 1.5 1.5 1.5 1.5 1.5 1.5 1.5 1.5 1.5 1.5 1.5 1.5 1.5 1.5 1.5 1.5 1.5],[1.9 1.9 1.9 1.9 1.9 1.9 1.9 1.9 1.9 1.9 1.9 1.9 1.9 1.9 1.9 1.9 1.9 1.9 1.9 1.9 1.9;1.9 1.9 1.9 1.9 1.9 1.9 1.9 1.9 1.9 1.9 1.9 1.9 1.9 1.9 1.9 1.9 1.9 1.9 1.9 1.9 1.9;1.9 1.9 1.9 1.9 1.9 1.9 1.9 1.9 1.9 1.9 1.9 1.9 1.9 1.9 1.9 1.9 1.9 1.9 1.9 1.9 1.9;1.9 1.9 1.9 1.9 1.9 1.9 1.9 1.9 1.9 1.9 1.9 1.9 1.9 1.9 1.9 1.9 1.9 1.9 1.9 1.9 1.9;1.9 1.9 1.9 1.9 1.9 1.9 1.9 1.9 1.9 1.9 1.9 1.9 1.9 1.9 1.9 1.9 1.9 1.9 1.9 1.9 1.9;1.9 1.9 1.9 1.9 1.9 1.9 1.9 1.9 1.9 1.9 1.9 1.9 1.9 1.9 1.9 1.9 1.9 1.9 1.9 1.9 1.9;1.9 1.9 1.9 1.9 1.9 1.9 1.9 1.9 1.9 1.9 1.9 1.9 1.9 1.9 1.9 1.9 1.9 1.9 1.9 1.9 1.9 ...(+1680 chars)])  CalLossMapData={'BaseCageProjectFileName','';'BaseMbcProjectFileName','';'TaskName','Calibrate Motor Loss Map';'ChildTasks',{{'DataName','';'TaskName','Import Loss Data'},{'TaskName','Generate Response Models'},{'TaskName','Generate Calibration'},{'TaskName','Update Block Parameters'}}}  CalLossWithTempMapData={}  aMode=6  RefBlkName='autolibmappedmotor/Mapped Motor'
  MaxAcceleration : Lookup_n-D  Commented=on  NumberOfTableDimensions=1  BreakpointsForDimension1=[0;5;20]  Table=[4;4;2]  ExtrapMethod=Clip  RemoveProtectionInput=on  UseLastTableValue=on  InternalRulePriority=Speed  RndMeth=Simplest
  MaximumNegativeJerk : Lookup_n-D  Commented=on  NumberOfTableDimensions=1  BreakpointsForDimension1=[0;5;20]  Table=[-5;-5;-2.5]  ExtrapMethod=Clip  RemoveProtectionInput=on  UseLastTableValue=on  InternalRulePriority=Speed  RndMeth=Simplest
  MaximumPositiveJerk : Lookup_n-D  Commented=on  NumberOfTableDimensions=1  BreakpointsForDimension1=[0;5;10]  Table=[1;1;4]  ExtrapMethod=Clip  RemoveProtectionInput=on  UseLastTableValue=on  InternalRulePriority=Speed  RndMeth=Simplest
  Memory : Memory  InitialCondition=(Init.VelocityVector(1) / Wheels.EffectiveRadius) * ones(1,4)  InheritSampleTime=on
  MinimumAcceleration : Lookup_n-D  Commented=on  NumberOfTableDimensions=1  BreakpointsForDimension1=[0;5;20]  Table=[-5;-5;-3.5]  ExtrapMethod=Clip  RemoveProtectionInput=on  UseLastTableValue=on  InternalRulePriority=Speed  RndMeth=Simplest
  Motor Coupling Dynamics : TransferFcn  Denominator=[0.01 1]
  Mux : Mux
  Mux1 : Mux
  Mux2 : Mux
  Product : Product  Inputs=3
  Product{1..6} (6 alike) : Product
  Rate Limiter : RateLimiter  RisingSlewLimit=500  FallingSlewLimit=-500  SampleTimeMode=inherited
  Rate Transition{,1,3..7} (7 alike) : RateTransition  Commented=on  Deterministic=off
  Rate Transition{8..13,16..18} (9 alike) : RateTransition  Deterministic=off
  Rate Transition14 : RateTransition  Commented=on
  Rate Transition15 : RateTransition  Commented=on
  Rate Transition19 : RateTransition  Deterministic=off  InitialCondition=Init.ElectircMotorSpeed
  Rate Transition2 : RateTransition  Commented=on  Deterministic=off  InitialCondition=[0 0 0]
  Rear Left Axle (1) Torsional Compliance : autolibsharedcoupling/Torsional Compliance  port_config=Simulink  extInfo=off  k=Drivetrain.RearAxleLeft.TorsionalStiffness  b=Drivetrain.RearAxleLeft.TorsionalDamping  theta_o=Init.RearAxleLeftDeflection  domega_o=Init.RearAxleLeftVelocityDifference  omega_c=Drivetrain.RearAxleLeft.DampingCutoffFreq  blkID=0  aMode=6
  Rear Right Axle (2) Torsional Compliance : autolibsharedcoupling/Torsional Compliance  port_config=Simulink  extInfo=off  k=Drivetrain.RearAxleRight.TorsionalStiffness  b=Drivetrain.RearAxleRight.TorsionalDamping  theta_o=Init.RearAxleRightDeflection  domega_o=Init.RearAxleRightVelocityDifference  omega_c=Drivetrain.RearAxleRight.DampingCutoffFreq  blkID=0  aMode=6
  Rotational Inertia : autolibsharedcoupling/Rotational Inertia  port_config=Simulink  extInfo=off  externJ=off  J=ElectricMotor.Inertia  b=ElectricMotor.TorsionalDamping  omega_o=Init.VelocityVector(1) / Wheels.EffectiveRadius * Drivetrain.RearDifferential.CarrierToDriveshaftRatio * Drivetrain.EngineToRearDriveshaftRatio  blkID=0  aMode=2
      settings: LibrarySourceBlock=vdynlib/Powertrain/Drivetrain/Couplings/Rotational Inertia
  Saturation Dynamic : simulink/Discontinuities/Saturation Dynamic  OutMin=[]  OutMax=[]  OutDataTypeStr=Inherit: Same as second input  OutDataType=fixdt(1, 16)  OutScaling=2^-10  DoSatur=off
  Scope : Scope  Commented=on
  Scope1 : Scope  NumInputPorts=5
  Scope2 : Scope  NumInputPorts=2
  Scope3 : Scope
  Scope4 : Scope
  Scope8 : Scope
  Selector : Selector  InputPortWidth=1  IndexOptions=Index vector (dialog)  Indices=[1 1]  OutputSizes=1
  Selector1 : Selector  InputPortWidth=4  IndexOptions=Index vector (dialog)  Indices=[3 4]  OutputSizes=1
  Selector2 : Selector  InputPortWidth=4  IndexOptions=Index vector (dialog)  Indices=[1]  OutputSizes=1
  Signal Specification : SignalSpecification  Unit=N*m
  Signal Specification1 : SignalSpecification  Unit=A
  Signal Specification2 : SignalSpecification  Unit=A
  Signal Specification3 : SignalSpecification  Unit=deg
  Simulation 3D Scene Configuration : sim3dlib/Simulation 3D Scene Configuration  Priority=0  Commented=on  ProjectFormat=Default Scenes  SceneDesc=Straight road  ProjectName=C:\Program Files\MATLAB\R2023b\toolbox\shared\sim3d_projects\automotive_project_windows\UE\WindowsNoEditor\VehicleSimulation.exe  ScenePath=/Game/Maps/HwStrght  EnableOpenDRIVE=off  vehTagList={'Scene Origin'}  vehTag=Scene Origin  FreeCameraInitialTranslation=[0, 0, 0]  FreeCameraDefaultInitialTranslation=[-6, 0, 2]  FreeCameraInitialRotation=[0, 0, 0]  FreeCameraDefaultInitialRotation=[0, -15, 0]  OpVisEn=off  Ts=.02  EnableWindow=on  EnableRemoteAccess=off  EnableWeather=off  SunAltitude=40.0  SunAzimuth=90  clouds=10  wind=1  fog=0  rain=0  EnableGeospatial=off  OriginHeight=200  OriginLatitude=40.744652  OriginLongitude=-73.988864  MapStyle=Aerial  AdditionalAssetIDs=[]  UseAdvancedSunSky=off  SolarTime=11  TimeZone=-5  Day=21  Month=9  Year=2022  UseDaylightSavingTime=on  DSTStartDay=10  DSTStartMonth=3  DSTEndDay=3  DSTEndMonth=11  DSTSwitchHour=2  sensorTag=MainCamera1  sensorId=1  sensorName=MainCamera1  mountLoc=Origin  offsetFlag=off  tmountOffset=[0, 0, 0]  rmountOffset=[0, 0, 0]  HorizontalResolution=1280  VerticalResolution=720  HorizontalFOV=60  mountPoint=[0 0 0]  mountOrientation=[0 0 0]  aMode=2  ID=1  GeoTrigger=Inactive
      settings: LibrarySourceBlock=vehdynlibsim3dcore/Simulation 3D Scene Configuration
  Simulation 3D Vehicle with Ground Following : sim3dautolib/Simulation 3D Vehicle with Ground Following VDBS  Priority=-1  Commented=on  PassVehMesh=Muscle car  MeshPath=/MathWorksSimulation/Vehicles/Muscle/Meshes/SK_MuscleCar.SK_MuscleCar  TrackWidth=1.9  WheelBase=3  WheelRadius=0.35  VehColor=Red  InitialPos=Init.PositionVector  InitialRot=Init.OrientationAngleVector  ActorName=SimulinkVehicle1  VehLightsControl=off  HeadlightColor=[ 1, 1, 1 ]  HighBeamIntensity=100000  LowBeamIntensity=60000  HighBeamConeAngle=1.22  LowBeamConeAngle=1.22  LeftHeadlightOrientation=[ 0, 0 ]  RightHeadlightOrientation=[ 0, 0 ]  BrakelightIntensity=200  ReverselightIntensity=500  SignallightIntensity=500  SignallightPeriod=1  SignalPulseWidth=50  SampleTime=-1  ActorType=SimulinkVehicle  ID=1  aMode=2  ActorTag=SimulinkVehicle1  CoordinateScheme=SAE
      settings: LibrarySourceBlock=vehdynlibsim3d/Simulation 3D Vehicle with Ground Following
  Solid Axle Suspension - Coil Spring : vehdynlibsuspension/Solid Axle Suspension - Coil Spring  NumAxl=1  NumWhlsByAxl=2  StrgEnByAxl=0  WhlNumVec="[1  2]"  AxleNumVec="[1  1]"  SuspTypesByAxle=[1]  SuspImage=suspsacoil.png  AxlIxx=Suspension.AxleAndWheelIxx  AxlM=Suspension.AxleAndWheelMass  TrackCoords=[0 0;Vehicle.TrackWidthRear*[-1 1]/2;0 0]  SuspCoords=[0 0;Vehicle.TrackWidthRear*[-1 1]/2;0 0]  KzWhlAxl=Suspension.AxleAndWheelComplianceConst  F0zWhlAxl=Suspension.AxleAndWheelCompiancePreload  CzWhlAxl=Suspension.AxleAndWheelDampingConst  IdealSuspEn=on  IdealSuspAxles=[1]  Kz=Suspension.SpringConstant  F0z=Suspension.SpringPreloadRear  Cz=Suspension.ShockDampingConstant  Hmax=Suspension.MaximumHeight  Toe=0.  RollStrgSlp=0.  ToeStrgSlp=0  Caster=0.  CasterHslp=0.  CasterStrgSlp=0.01  Camber=0.  CamberHslp=0.  CamberStrgSlp=0.01  StrgHgtSlp=0.1432  MappedSuspEn=off  MappedSuspAxles="[1  2]"  f_susp_axl_bp=[1 2]  f_susp_dz_bp=[-0.15 -0.14 -0.13 -0.12 -0.11 -0.10 -0.09 -0.08 -0.07 -0.06 -0.05 -0.04 -0.03 -0.02 -0.01 0.00 0.01 0.02 0.03 0.04 0.05 0.06 0.07 0.08 0.09 0.10 0.11 0.12 0.13 0.14 0.15]  f_susp_dzdot_bp=[-0.15 -0.14 -0.13 -0.12 -0.11 -0.10 -0.09 -0.08 -0.07 -0.06 -0.05 -0.04 -0.03 -0.02 -0.01 0.00 0.01 0.02 0.03 0.04 0.05 0.06 0.07 0.08 0.09 0.10 0.11 0.12 0.13 0.14 0.15]  f_susp_fmz=zeros(31,31,61,2,4)  f_susp_geom=zeros(31,61,2,3)  f_susp_strgdelta_bp=[-30,-29,-28,-27,-26,-25,-24,-23,-22,-21,-20,-19,-18,-17,-16,-15,-14,-13,-12,-11,-10,-9,-8,-7,-6,-5,-4,-3,-2,-1,0,1,2,3,4,5,6,7,8,9,10,11,12,13,14,15,16,17,18,19,20,21,22,23,24,25,26,27,28,29,30]
  SteeringWheelAngle : Constant  Value=0
  Step : Step  SampleTime=0
  Suspension Adapter : Subsystem
  Suspension Bus Creator : Subsystem
  Suspension to Chasiss Transforms : Subsystem
  Switch : Switch  Criteria=u2 > Threshold  SaturateOnIntegerOverflow=off  InputSameDT=off
  Terminator{,1..32,38} (34 alike) : Terminator
  Terminator{33..37} (5 alike) : Terminator  Commented=on
  Three-axis Inertial Measurement Unit : vehdynlibsens/Three-axis Inertial Measurement Unit  Commented=on  units=Metric (MKS)  imu=[0 0 0]  i_Ts=0  dtype_a=off  w_a=190  z_a=0.707  a_sf_cc=[1 0 0; 0 1 0; 0 0 1]  a_bias=[0 0 0]  a_sat="[-inf  -inf  -inf  inf inf inf]"  dtype_g=off  w_g=190  z_g=0.707  g_sf_cc=[1 0 0; 0 1 0; 0 0 1]  g_bias=[0 0 0]  g_sens=[0 0 0]  g_sat="[-inf  -inf  -inf  inf inf inf]"  i_rand=on  i_seeds=[23093 23094 23095 23096 23097 23098]  i_pow=[0.001 0.001 0.001 0.0001 0.0001 0.0001]  aMode=2
  Tire2Veh : Subsystem
  Triggered Subsystem : Subsystem  TreatAsAtomicUnit=on
  Unit Conversion : UnitConversion  Commented=on
  Unit Conversion1 : UnitConversion
  Valve : autolibutils/Cont LPF  wc=Brakes.CutoffFreq  AbsoluteTolerance=auto  aMode=2
  Vehicle Body 6DOF : vehdynlibeom/Vehicle Body 6DOF  extPos=on  extVel=on  extEuler=on  extRotRate=on  htchFMode=off  htchMMode=off  m=Vehicle.Mass  a=Vehicle.CG.LongDistFrontAxle  b=Vehicle.CG.LongDistRearAxle  d=Vehicle.CG.LateralOffsetFromCenterline  h=Vehicle.CG.VerticalOffsetFromAxlePlane  dh=1  hl=0  hh=0.1  Xe_o=Init.PositionVector  xbdot_o=Init.VelocityVector  eul_o=Init.OrientationAngleVector  p_o=Init.AngularVelocityVector  Iveh=[Vehicle.InertiaRoll 0 0; 0 Vehicle.InertiaPitch 0; 0 0 Vehicle.InertiaYaw]  w=[Vehicle.TrackWidthFront Vehicle.TrackWidthRear]  z1m=0  z1R=[-.25,.125,.15]  z1I=[1.4,-.2,.1;-.2,1.4,.1;.1,.1,2.25].*0  z2m=0  z2R=[1.4,0,.8]  z2I=[1.4,-.2,.1;-.2,1.4,.1;.1,.1,2.25].*0  z3m=0  z3R=[.75,-.5,.4]  z3I=[5,-.1,-2;-2,9,.1;-.1,.1,6].*0  z4m=0  z4R=[.75,.5,.4]  z4I=[5,-.1,-2;-2,9,.1;-.1,.1,6].*0  z5m=0  z5R=[1.25,-.5,.4]  z5I=[5,-.1,-2;-2,9,.1;-.1,.1,6].*0  z6m=0  z6R=[1.25,-.5,.4]  z6I=[5,-.1,-2;-2,9,.1;-.1,.1,6].*0  z7m=0  z7R=[2,0,.25]  z7I=[1.4,-.2,.1;-.2,1.4,.1;.1,.1,2.25].*0  Af=Vehicle.DragAreaLongitudinal  Cd=Vehicle.DragCoefficientLongitudinal  Cl=Vehicle.LiftCoefficientLongitudinal  Cpm=Vehicle.DragPitchMoment  beta_w=Vehicle.RelativeWindAngleVector  Cs=Vehicle.SideForceCoeffVector  Cym=Vehicle.YawMomentCoeffVector  Pabs=Env.AbsolutePressure  extTamb=off  Tair=Env.AirTemperature  g=Env.Gravity  xdot_tol=.1  longOff=0  latOff=0  vertOff=0  wrapAng=off  aMode=2
  Wheel Adapter : Subsystem
  XY Graph : Record  FileSettingsInternal="{\"entries\":[{\"content\":{\"excelSettings\":{\"content\":{},\"type\":\"Streamout.ExcelSettings\"}},\"type\":\"Streamout.FileSettingStorage\",\"uuid\":\"\"}],\"packageUris\":[\"http:\\/\\/schema.mathworks.com\\/mf0\\/streamout_blocks\\/R2020a\"],\"version\":\"1.0\"}"  Layout=[1 1]  SignalsInternal="{\"entries\":[{\"content\":{\"signals\":[{\"content\":{\"blockPath\":[],\"dimensions\":[1],\"domain\":\"\",\"lineColor\":\"#0072bd\",\"port\":1,\"sid\":[\"\"],\"signalID\":1,\"signalName\":\"<X>\"},\"type\":\"RecordBlkView.Signal\",\"uuid\":\"\"},{\"content\":{\"blockPath\":[],\"dimensions\":[1],\"domain\":\"\",\"lineColor\":\"#d95319\",\"port\":2,\"sid\":[\"\"],\"signalID\":2,\"signalName\":\"Gain\"},\"type\":\"RecordBlkView.Signal\",\"uuid\":\"\"}]},\"type\":\"RecordBlkView.InputSignals\",\"uuid\":\"\"}],\"packageUris\":[\"http:\\/\\/schema.mathworks.com\\/mf0\\/streamout_blocks\\/R2020a\"],\"version\":\"1.0\"}"  VisualizationBindings="{\"xyplotplugin\":{\"info\":[{\"series\":[],\"subplotID\":1}]}}"  CompatibilityTag=XY
  independent Suspensions - MacPherson : vehdynlibsuspension/Independent Suspension - MacPherson  ActiveDampEn=off  NumAxl=1  NumWhlsByAxl=2  StrgEnByAxl=1  AntiSwayEnByAxl=1  WhlNumVec="[1  2]"  AxleNumVec="[1  1]"  SuspTypesByAxle=[1]  SuspImage=suspmacp.png  IdealSuspEn=on  IdealSuspAxles=[1]  Kz=Suspension.SpringConstant  F0z=Suspension.SpringPreloadFront  Cz=Suspension.ShockDampingConstant  Hmax=Suspension.MaximumHeight  f_act_susp_cz=[10000 10000;10000 10000]  f_act_susp_duty_bpt=[0 1]  f_act_susp_zdot_bpt=[-1 1]  Toe=0  RollStrgSlp=0.  ToeStrgSlp=0.  Caster=0.  CasterHslp=0.  CasterStrgSlp=0.  Camber=-0.5*pi/180*0  CamberHslp=0.  CamberStrgSlp=0.  StrgHgtSlp=0.1432  MappedSuspEn=off  MappedSuspAxles="[1  2]"  f_susp_axl_bp=[1 2]  f_susp_dz_bp=[-0.15 -0.14 -0.13 -0.12 -0.11 -0.10 -0.09 -0.08 -0.07 -0.06 -0.05 -0.04 -0.03 -0.02 -0.01 0.00 0.01 0.02 0.03 0.04 0.05 0.06 0.07 0.08 0.09 0.10 0.11 0.12 0.13 0.14 0.15]  f_susp_dzdot_bp=[-0.15 -0.14 -0.13 -0.12 -0.11 -0.10 -0.09 -0.08 -0.07 -0.06 -0.05 -0.04 -0.03 -0.02 -0.01 0.00 0.01 0.02 0.03 0.04 0.05 0.06 0.07 0.08 0.09 0.10 0.11 0.12 0.13 0.14 0.15]  f_susp_fmz=zeros(31,31,61,2,4)  f_susp_geom=zeros(31,61,2,3)  f_susp_strgdelta_bp=[-30,-29,-28,-27,-26,-25,-24,-23,-22,-21,-20,-19,-18,-17,-16,-15,-14,-13,-12,-11,-10,-9,-8,-7,-6,-5,-4,-3,-2,-1,0,1,2,3,4,5,6,7,8,9,10,11,12,13,14,15,16,17,18,19,20,21,22,23,24,25,26,27,28,29,30]  AntiSwayR=0.2  AntiSwayNtrlAng=0.5236  AntiSwayTrsK=8e+02
  Out1 : Outport
  sri_val : Outport  Port=2
  Acc from Control : Outport  Port=3
  wires:
  AccelerationToTrq/3(IntendedTrq[Nm]) -> Scope1/2  "IntendedTorque(NoLimit)"
  [HV_speed] -> Scope1/4  "HVSpeed"
  [EngineSpeedFbdk] -> Gain1/1  "EngineSpeed[rpm]"
  Memory/1 -> Selector1/1
  Bus Selector15/2 -> Gain/1, Simulation 3D Vehicle with Ground Following/2  "<Y>"
  Wheel Adapter/11(WhlAng) -> Tire2Veh/4(WhlAng)
  Rear Left Axle (1) Torsional Compliance/2 -> Mux/3  "RL"
  Rate Transition13/1 -> DrivetrainControlUnit/8(BMSChrgCurrLmt)
  Constant24/1 -> Product1/2
  Bus Selector1/2 -> Rate Transition/1  "<BrkPrs>"
  Constant31/1 -> DrivetrainControlUnit/2(BcuBrkPrsCmd)
  Lateral Driver/2 -> Terminator36/1
  Mapped Motor/3 -> Motor Coupling Dynamics/1
  Rate Transition19/1 -> 1-D Lookup Table/1
  Bus Selector16/1 -> Longitudinal Driver/3  "<Grade>"
  DrivetrainControlUnit/1(EMTrqCmd) -> Rate Limiter/1
  DrivetrainControlUnit/2(DcuBrkPrsCmd) -> Terminator38/1
  Selector/1 -> Demux2/1
  Wheel Adapter/12(WhlCmb) -> Tire2Veh/5(WhlCmb)
  Bus Selector21/1 -> Rate Transition17/1  "<Fx>"
  Solid Axle Suspension - Coil Spring/6 -> Terminator10/1
  [HV_speed] -> AccelerationToTrq/2(LongVehSpd[m/s])
  [BrakeCommand] -> Dead Zone/1
  RelativeVelocity/1 -> Adaptive Cruise Control System1/5
  Constant36/1 -> Product2/1
  independent Suspensions - MacPherson/4 -> Terminator11/1
  From11/1 -> Bus Selector8/1
  Rate Limiter/1 -> [TorqueCommand]
  Product3/1 -> Rotational Inertia/1
  Constant14/1 -> Bus Creator2/1  "DCM"
  Product5/1 -> First Order Hold/1, Scope2/2
  Lateral Driver/1 -> Terminator37/1
  Mapped Motor/2 -> Terminator32/1
  [EngineSpeedFbdk] -> Rate Transition19/1
  Bus Selector10/1 -> Memory/1  "<Omega>"
  Constant/1 -> Signal Specification/1
  Product4/1 -> [EngineSpeedFbdk], Mapped Motor/2
  Bus Selector3/1 -> independent Suspensions - MacPherson/7  "<VehPFront>"
  Rear Right Axle (2) Torsional Compliance/2 -> Mux/4  "RR"
  Constant37/1 -> Product4/1, Product3/2
  Saturation Dynamic/1 -> Switch/3, Scope1/3, Acc from Control/1  "IntendedLongAcceleration"
  Combined Slip Wheel 2DOF/4 -> Terminator28/1
  Bus Selector7/4 -> Solid Axle Suspension - Coil Spring/4  "<FxRear>"
  AccelerationToTrq/2(IntendedMainBrakePress[Pa]) -> Scope2/1, Product5/1
  Constant33/1 -> AccelerationToTrq/13(MaxMainBrakePress[Pa])
  Product2/1 -> AccelerationToTrq/14(BrakeTrqPressRatio[m**3])
  AccelerationToTrq/1(IntendedDriveTrq[Nm]) -> DrivetrainControlUnit/9(IntendedDriveTrq[Nm])
  Constant35/1 -> AccelerationToTrq/12(StandstillSwitch[0;1])
  1-D Lookup Table/1 -> AccelerationToTrq/11(FullAccPedalTrq[Nm])
  Constant27/1 -> AccelerationToTrq/9(TorqueRatio[-])
  Constant26/1 -> AccelerationToTrq/5(EngInrt[kg*m**2])
  Constant25/1 -> AccelerationToTrq/4(OverallMass[kg])
  Selector2/1 -> AccelerationToTrq/6(WheelRotAxisInrt[kg*m**2])
  Bus Selector18/2 -> Lateral Driver/3  "<Y>"
  Product1/1 -> AccelerationToTrq/3(UnloadedTireRadius[m])
  Rate Transition17/1 -> AccelerationToTrq/8(AeroFrc(VehSys)[N])
  Suspension Adapter/2(VehSusp) -> Bus Selector3/1, Bus Selector4/1
  FiveSteteABS-TCS/3(TCSFlag) -> Terminator34/1
  Three-axis Inertial Measurement Unit/2 -> Bus Creator1/2  "pqr"
  Suspension Bus Creator/1(Suspension) -> Suspension to Chasiss Transforms/1(Suspension), [SuspensionFbdk]
  From18/1 -> Bus Selector17/1
  Suspension to Chasiss Transforms/1(FsB) -> Vehicle Body 6DOF/1
  Constant3/1 -> Mux2/3, Mux2/4
  Solid Axle Suspension - Coil Spring/1 -> Bus Creator/2  "Rear"
  First Order Hold/1 -> [BrakeCommand]
  Wheel Adapter/1(BrkPrs) -> Combined Slip Wheel 2DOF/1
  Bus to Vector1/1 -> Three-axis Inertial Measurement Unit/2
  Dead Zone/1 -> Valve/1
  Constant13/1 -> Bus Creator2/5  "Grade"
  Bus Selector3/2 -> independent Suspensions - MacPherson/8  "<VehVFront>"
  Rear Left Axle (1) Torsional Compliance/1 -> Limited Slip Differential/2
  Bus Selector7/3 -> Solid Axle Suspension - Coil Spring/3  "<zdotRear>"
  Wheel Adapter/4(Vy) -> Combined Slip Wheel 2DOF/4
  Rate Transition11/1 -> DrivetrainControlUnit/6(BattPackVolt)
  Solid Axle Suspension - Coil Spring/3 -> Terminator15/1
  Bus Selector2/1 -> Bus to Vector/1
  Limited Slip Differential/2 -> Driveshaft Compliance/2
  Demux1/2 -> Rear Right Axle (2) Torsional Compliance/2
  Tire2Veh/7(SuspWhlPz) -> Terminator24/1
  Bus Creator2/1 -> [ENV]
  independent Suspensions - MacPherson/6 -> Terminator7/1
  Bus to Vector2/1 -> Three-axis Inertial Measurement Unit/3
  Mapped Motor/1 -> Terminator31/1
  Tire2Veh/4(FrntAxlF) -> Terminator21/1
  [VehicleFbdk] -> Bus Selector15/1
  Tire2Veh/8(SuspWhlVz) -> Wheel Adapter/6(zdot)  "zdot"
  Suspension Adapter/1(WheelsSusp) -> Bus Selector7/1, Bus Selector/1
  Bus Selector4/2 -> Solid Axle Suspension - Coil Spring/8  "<VehVRear>"
  Tire2Veh/5(RearAxlF) -> Terminator22/1
  Selector1/1 -> Demux1/1
  Bus Selector5/1 -> Bus to Vector1/1
  Bus Selector19/1 -> Rate Transition16/1  "<xdot>"
  Combined Slip Wheel 2DOF/6 -> Terminator18/1
  Constant30/1 -> Product1/1
  Mux1/1 -> Suspension Adapter/1(Steer)
  Constant23/1 -> Selector2/1
  independent Suspensions - MacPherson/3 -> Terminator12/1
  Constant4/1 -> Product/2
  Rate Transition5/1 -> Rate Transition7/1
  Bus Selector17/1 -> Rate Transition14/1  "<xdot>"
  Bus Selector/1 -> independent Suspensions - MacPherson/1  "<zFront>"
  [VehicleFbdk] -> Bus Selector21/1
  Bus Selector20/1 -> Rate Transition18/1
  Wheel Adapter/9(Fext) -> Combined Slip Wheel 2DOF/9, Tire2Veh/3(Fz)
  Wheel Adapter/6(YawRate) -> Combined Slip Wheel 2DOF/6
  Vehicle Body 6DOF/3 -> Terminator1/1
  [WheelFbdk] -> Bus Selector20/1
  Demux1/1 -> Rear Left Axle (1) Torsional Compliance/2
  Bus Selector7/6 -> Solid Axle Suspension - Coil Spring/6  "<MRear>"
  Rate Transition2/1 -> FiveSteteABS-TCS/3(Acc)
  Demux2/2 -> Mux/2  "FR"
  From20/1 -> Bus Selector18/1
  Suspension to Chasiss Transforms/3(Fext) -> Vehicle Body 6DOF/3
  Constant12/1 -> Lateral Driver/1
  Combined Slip Wheel 2DOF/5 -> Terminator17/1
  Bus Selector11/1 -> Rate Transition8/1  "<xdot>"
  Signal Specification3/1 -> Unit Conversion1/1
  [WheelFbdk] -> Bus Selector10/1
  Rate Transition14/1 -> Longitudinal Driver/2
  [VehicleFbdk] -> Bus Selector11/1
  Constant29/1 -> AccelerationToTrq/10(ZeroAccPedalTrq[Nm])
  Bus Selector18/5 -> Lateral Driver/6  "<r>"
  Bus Selector18/4 -> Lateral Driver/5  "<psi>"
  Bus Selector18/3 -> Lateral Driver/4  "<ydot>"
  Bus Selector9/1 -> independent Suspensions - MacPherson/9  "<StrgAngFront>"
  Rate Transition15/1 -> Lateral Driver/2
  Solid Axle Suspension - Coil Spring/5 -> Terminator9/1
  From17/1 -> Bus Selector16/1
  Bus Selector/3 -> independent Suspensions - MacPherson/3  "<zdotFront>"
  Bus Selector12/2 -> Wheel Adapter/4(Friction)  "<Friction>"
  Bus Selector18/1 -> Rate Transition15/1  "<xdot>"
  Rate Transition4/1 -> FiveSteteABS-TCS/2(DecelFdbk)
  Longitudinal Driver/2 -> Rate Transition3/1, Rate Transition6/1
  Wheel Adapter/2(AxlTrq) -> Combined Slip Wheel 2DOF/2
  Bus Selector12/1 -> Wheel Adapter/3(Ground Input)  "<Ground>"
  Limited Slip Differential/4 -> Rear Right Axle (2) Torsional Compliance/1
  [TorqueCommand] -> Scope1/1  "TorqueCmd(Engine)"
  Vehicle Body 6DOF/4 -> Terminator2/1
  Driveshaft Compliance/2 -> Limited Slip Differential/1
  Constant18/1 -> Mux1/3, Mux1/4
  Bus Selector7/5 -> Solid Axle Suspension - Coil Spring/5  "<FyRear>"
  From19/1 -> Bus Selector6/1, Bus Selector2/1, Bus Selector5/1
  Bus Selector15/3 -> Simulation 3D Vehicle with Ground Following/3  "<psi>"
  Constant5/1 -> [BatteryVoltage], Mapped Motor/1
  Suspension Adapter/3(SteeringAngles) -> Bus Selector9/1
  Combined Slip Wheel 2DOF/1 -> [WheelFbdk], Tire2Veh/1(Wheels)  "TireFrame"
  independent Suspensions - MacPherson/5 -> Terminator8/1
  Constant1/1 -> Vehicle Body 6DOF/4
  Kinematic Steering/1 -> Terminator30/1
  Vehicle Body 6DOF/5 -> Terminator3/1
  Vehicle Body 6DOF/7 -> Terminator5/1
  Wheel Adapter/8(Gnd) -> Combined Slip Wheel 2DOF/8
  Bus Selector/5 -> independent Suspensions - MacPherson/5  "<FyFront>"
  Solid Axle Suspension - Coil Spring/2 -> Terminator14/1
  [EngineSpeedFbdk] -> Rate Transition9/1
  Tire2Veh/6(<Mz>) -> Terminator23/1
  Rate Transition9/1 -> DrivetrainControlUnit/4(EMSpd)
  Longitudinal Driver/3 -> Rate Transition4/1
  independent Suspensions - MacPherson/1 -> Bus Creator/1  "Front"
  Bus Selector4/1 -> Solid Axle Suspension - Coil Spring/7  "<VehPRear>"
  Bus Selector15/1 -> Simulation 3D Vehicle with Ground Following/1, XY Graph/1  "<X>"
  Bus Selector/2 -> independent Suspensions - MacPherson/2  "<ReFront>"
  Wheel Adapter/7(Prs) -> Combined Slip Wheel 2DOF/7
  Vehicle Body 6DOF/1 -> Out1/1, [VehicleFbdk], Suspension to Chasiss Transforms/2(VehFdbk)
  Demux2/1 -> Mux/1  "FL"
  Gain/1 -> XY Graph/2
  RelDist/1 -> MATLAB Function1/7(RelDist), Adaptive Cruise Control System1/4
  Constant32/1 -> Product2/2
  Mux2/1 -> Product/1
  Kinematic Steering/2 -> Mux1/1
  Signal Specification1/1 -> Rate Transition12/1
  Bus Creator/1 -> Suspension Bus Creator/2(SuspensionInfo)
  Limited Slip Differential/3 -> Rear Left Axle (1) Torsional Compliance/1
  Wheel Adapter/10(ScaleFctrs) -> Combined Slip Wheel 2DOF/10
  [ENV] -> Bus Selector14/1
  SteeringWheelAngle/1 -> Signal Specification3/1
  Tire2Veh/1(Wheel) -> Terminator29/1
  Combined Slip Wheel 2DOF/7 -> Terminator19/1
  Bus Selector/6 -> independent Suspensions - MacPherson/6  "<MFront>"
  Product/1 -> Wheel Adapter/5(Brake Press)
  Driveshaft Compliance/1 -> Rotational Inertia/2
  [VehicleFbdk] -> Tire2Veh/2(Veh)
  Motor Coupling Dynamics/1 -> Product3/1  "EMTrq"
  Bus Selector14/1 -> Vehicle Body 6DOF/5  "<WindXYZ>"
  Bus Selector/4 -> independent Suspensions - MacPherson/4  "<FxFront>"
  Combined Slip Wheel 2DOF/2 -> Terminator26/1
  [BatteryVoltage] -> Rate Transition11/1
  Bus Selector8/1 -> Bus to Vector3/1
  Wheel Adapter/3(Vx) -> Combined Slip Wheel 2DOF/3
  Rotational Inertia/1 -> Driveshaft Compliance/1, Product4/2
  Bus to Vector3/1 -> Rate Transition2/1
  Rear Right Axle (2) Torsional Compliance/1 -> Limited Slip Differential/3
  Constant28/1 -> DrivetrainControlUnit/1(AccelPdl)
  Bus Selector6/1 -> Bus to Vector2/1
  Signal Specification2/1 -> Rate Transition13/1
  [TorqueCommand] -> Mapped Motor/3
  FiveSteteABS-TCS/2(ABSFlag) -> Terminator33/1
  Bus Selector1/1 -> Rate Transition1/1  "<Omega>"
  Solid Axle Suspension - Coil Spring/4 -> Terminator16/1
  Constant2/1 -> Mux2/2, Mux2/1
  Rate Transition10/1 -> DrivetrainControlUnit/5(BMSSOC)
  FiveSteteABS-TCS/1(BrkPrsCmd) -> Rate Transition5/1
  Constant6/1 -> Rate Transition10/1  "SOC_CC"
  [ENV] -> Bus Selector13/1
  Rate Transition3/1 -> FiveSteteABS-TCS/1(AccelFdbk)
  Valve/1 -> Product/3
  Constant20/1 -> Adaptive Cruise Control System1/2
  [SteeringWheelCommand] -> Kinematic Steering/1
  Rate Transition8/1 -> DrivetrainControlUnit/3(VehSpdFdbk)
  Mux/1 -> Wheel Adapter/2(Axle Torque)
  From5/1 -> Bus Selector1/1
  Bus Creator1/1 -> Goto6/1  "IMU"
  Unit Conversion/1 -> Three-axis Inertial Measurement Unit/1
  Three-axis Inertial Measurement Unit/1 -> Bus Creator1/1  "Acc"
  Constant16/1 -> Bus Creator2/3  "Ground"
  [VehicleFbdk] -> Suspension Adapter/2(Vehicle)
  Vehicle Body 6DOF/2 -> Terminator/1
  [VehicleFbdk] -> Suspension Bus Creator/1(Vehicle)
  Unit Conversion1/1 -> [SteeringWheelCommand]
  Combined Slip Wheel 2DOF/3 -> Terminator27/1
  Rate Transition/1 -> FiveSteteABS-TCS/5(BrkPrs)
  Constant9/1 -> Three-axis Inertial Measurement Unit/4
  [SuspensionFbdk] -> Wheel Adapter/1(Suspension)
  Vehicle Body 6DOF/6 -> Terminator4/1
  Bus to Vector/1 -> Unit Conversion/1
  [ENV] -> Bus Selector12/1
  Constant15/1 -> Bus Creator2/2  "Friction"
  Rate Transition1/1 -> FiveSteteABS-TCS/4(Omega)
  Bus Selector15/4 -> Scope/1  "<xdot>"
  Combined Slip Wheel 2DOF/8 -> Terminator20/1
  Suspension to Chasiss Transforms/2(MsB) -> Vehicle Body 6DOF/2
  Rate Transition12/1 -> DrivetrainControlUnit/7(BMSDischrgCurrLmt)
  Signal Specification/1 -> Selector/1  "FR"
  Bus Selector13/1 -> Wheel Adapter/7(DCM), Tire2Veh/6(DCM)  "<DCM>"
  Kinematic Steering/3 -> Mux1/2
  Bus Selector7/1 -> Solid Axle Suspension - Coil Spring/1  "<zRear>"
  Constant10/1 -> Three-axis Inertial Measurement Unit/5
  Tire2Veh/3(Omega) -> Terminator25/1
  Bus Selector7/2 -> Solid Axle Suspension - Coil Spring/2  "<ReRear>"
  Constant8/1 -> Signal Specification2/1  "ChargeCurrentLimit"
  Tire2Veh/2(Wheels2Susp) -> Suspension Bus Creator/3(Wheels), Suspension Adapter/3(Wheels)  "Wheels"
  Wheel Adapter/5(Camber) -> Combined Slip Wheel 2DOF/5
  [VehicleFbdk] -> Bus Selector19/1
  Longitudinal Driver/1 -> Terminator35/1
  Rate Transition16/1 -> [HV_speed], Adaptive Cruise Control System1/3
  Constant7/1 -> Signal Specification1/1  "DischargeCurrentLimit"
  Constant11/1 -> Longitudinal Driver/1
  Limited Slip Differential/1 -> Terminator6/1
  Constant17/1 -> Bus Creator2/4  "WindXYZ"
  Rate Transition18/1 -> AccelerationToTrq/7(TireMaxRollResistanceTrq[Nm])
  independent Suspensions - MacPherson/2 -> Terminator13/1
  Constant21/1 -> Product5/2
  Gain1/1 -> Scope1/5
  [HV_speed] -> 1-D Lookup Table1/1, MinimumAcceleration/1, MaximumNegativeJerk/1, MaximumPositiveJerk/1, MaxAcceleration/1
  1-D Lookup Table1/1 -> Saturation Dynamic/1  "IntendedLongAcceleration"
  Adaptive Cruise Control System1/1 -> Saturation Dynamic/2  "Acceleration of ego"
  Constant22/1 -> Saturation Dynamic/3
  MATLAB Function1/1(RefSpeedMax) -> Scope8/1
  Constant40/1 -> MATLAB Function1/1(RefSpeed)
  [HV_speed] -> Display/1, MATLAB Function1/2(v_HV)
  PDR/1 -> MATLAB Function1/4(pdr)
  Constant38/1 -> MATLAB Function1/5(lat)
  Constant39/1 -> MATLAB Function1/6(sri_target)
  MATLAB Function1/2(sri_val) -> sri_val/1, Scope3/1
  u/1 -> Display1/1, MATLAB Function1/3(v_RV)  "RelativeVelocity"
  MATLAB Function1/3(Headway) -> Scope4/1
  Constant19/1 -> Adaptive Cruise Control System1/1
  TTC/1 -> Compare To Constant1/1
  Switch/1 -> Display3/1, AccelerationToTrq/1(IntendedLongAcc[m/s**2])
  Compare To Constant1/1 -> Enabled Subsystem/Enable
  Clock/1 -> Product6/2
  Constant41/1 -> Enabled Subsystem/1(In1)
  Enabled Subsystem/1(Out1) -> Display2/1, Switch/2
  Constant34/1 -> Switch/1
